simulink model "METI_Thermal_ver01_Jmaab_2018b_Intg_Mref"  (R2018b)
settings: Solver=ode8  StartTime=0  StopTime=end_time  FixedStep=sampling_time  RelTol=1e-3
PreLoadFcn:
  | %init_setting;
values from neighbouring files (symbols this model uses):
  degC2K = 273.15    [METI_TRAMI_Thermal_ver01_Jmaab_PreLoad.m]    (also in init_setting_METI.m)
  K2degC = -273.15    [METI_TRAMI_Thermal_ver01_Jmaab_PreLoad.m]    (also in init_setting_METI.m)
  sampling_time = 0.0025    [METI_TRAMI_Thermal_ver01_Jmaab_PreLoad.m]
undefined symbols (not defined in the file or in its folder): ACC_D_Gain, ACC_I_Gain, ACC_P_Gain, ALT_CNT_ALT_OFF_RPM_HYS_rpm, ALT_CNT_ALT_ON_RPM_HYS_rpm, ALT_CNT_Alter_V_BASE_V, ALT_CNT_Alter_V_Kaisei_V, ALT_CNT_flag_disable_kaisei, ALT_CNT_V_Battely_Kudo_V, ALT_PNT_ALT_GDCurrent_A, ALT_PNT_ALT_GDVolt_V, ALT_PNT_Alter_limit_Current_V_table, ALT_PNT_Alter_limit_Current_V_table_x_rpm, ALT_PNT_Alter_trq_Nm_map, ALT_PNT_Alter_trq_Nm_map_x_rpm, ALT_PNT_Alter_trq_Nm_map_y_Current_A, ALT_PNT_Alter_trq_Nm_map_z_Volt_tgt_V, ALT_PNT_eta_pulley_alt, ALT_PNT_Gain_Alt_v_del, ALT_PNT_ratio_pulley_alt, ALT_PNT_Tau_Alternator_V_tgt_s, ALT_PNT_trq_alter_output_LL_Nm, BK_PNT_Pow_UL, BK_PNT_Tau_brake, Brk_LL, Brk_PGain, Brk_UL, BT_PNT_Lo_Capa_lo_batt_F, BT_PNT_Lo_ocv_SOC_lo_batt_OCV_V_table, BT_PNT_Lo_ocv_SOC_lo_batt_OCV_V_table_x_SOC, BT_PNT_Lo_R_lo_batt_ohm, BT_PNT_Lo_SOC_MAX_lo_batt, BT_PNT_Lo_SOC_MIN_lo_batt, BT_PNT_Lo_SOC_START_lo_batt, BT_PNT_Lo_V_start_ocv, DF_PNT_DF_gear, DF_PNT_Outtemp_degC, Driver_Brake_Const1, Driver_Brake_Const3, Driver_Brake_Switch_Const2, Driver_Brk_sh, drivmode_ACC, drivmode_CONST, drivmode_GensokuKaisei, drivmode_GensokuRikko, drivmode_STOP, EL_PNT_R_bodyelec_lo_ohm, ENG_CNT_acc_idlestop, ENG_CNT_Accel_LL, ENG_CNT_Accel_UL, ENG_CNT_brak_idlestop, ENG_CNT_flag_idle_stop_exe, ENG_CNT_gain_p_per_isc, ENG_CNT_IdleSpeed, ENG_CNT_IdleSpeed_Const, ENG_CNT_IdleStop_flag_const, ENG_CNT_omg_eng_fuelcut_rpm, ENG_CNT_per_isc_max, ENG_CNT_per_isc_min, ENG_CNT_per_throttle_fuelcut ... (+82)
libraries: METI_Lib_vehicle_model x18, simulink x3, AZAPA_Lib_vehicle_model x1
(part 3 of 3)

== system METI_Thermal_ver01_Jmaab_2018b_Intg_Mref/Vehicle/CNT/ENG_CNT/ENG_Cntrl/Starter ==
  note: サンプリング時間
  note: 時間リセット
  note: アイドリングフラグがON→OFFに
      | 切り替わり時スターターON開始
  note: スタータ開始時間
  note: スタータ開始時間から
      | ある時間超えたらOFF
  note: アイドリングフラグがON→OFFに切り替わり時スターターON開始.ある時間を超えたらOFF
  flag_idlestop : Inport
  n_eng_rpm : Inport  Port=2
  Constant2 : Constant  Value=ENG_CNT_Starter_timer_Const_s
  Constant4 : Constant  Value=sampling_time
  Constant5 : Constant  Value=0
  Constant6 : Constant  Value=OFF
  Constant7 : Constant  Value=ON
  IdleSpeed : Constant  Value=ENG_CNT_IdleSpeed_Const/2
  Logical Operator : Logic  Inputs=3  AllPortsSameDT=off  OutDataTypeStr=boolean
  Logical Operator1 : Logic  Operator=NOT  AllPortsSameDT=off  OutDataTypeStr=boolean
  Memory : Memory  InitialCondition=1000
  Memory1 : Memory  InheritSampleTime=on
  Relational Operator1 : RelationalOperator  Operator=<=  OutDataTypeStr=boolean  RndMeth=Nearest
  Relational Operator2 : RelationalOperator  Operator=<  OutDataTypeStr=boolean  RndMeth=Nearest
  Sum5 : Sum  Inputs=|++
  Switch3 : Switch  Criteria=u2 > Threshold  Threshold=0.5
  Switch4 : Switch  Criteria=u2 > Threshold  Threshold=0.5
  flag_ON_Starter : Outport
  wires:
  Switch4/1 -> flag_ON_Starter/1
  Memory/1 -> Sum5/2
  Constant4/1 -> Sum5/1
  Constant5/1 -> Switch3/1
  Sum5/1 -> Switch3/3
  Switch3/1 -> Relational Operator1/1, Memory/1
  Memory1/1 -> Logical Operator/2
  Logical Operator1/1 -> Logical Operator/1
  flag_idlestop/1 -> Memory1/1, Logical Operator1/1
  Logical Operator/1 -> Switch3/2
  Constant2/1 -> Relational Operator1/2
  Relational Operator1/1 -> Switch4/2
  Constant7/1 -> Switch4/1
  Constant6/1 -> Switch4/3
  n_eng_rpm/1 -> Relational Operator2/1
  IdleSpeed/1 -> Relational Operator2/2
  Relational Operator2/1 -> Logical Operator/3

== system METI_Thermal_ver01_Jmaab_2018b_Intg_Mref/Vehicle/CNT/ENG_CNT/ENG_Cntrl/Water_Pump_Control ==
  T_ENGTH_PNT_Coolant_dC : Inport
  1-D Lookup Table1 : Lookup_n-D  NumberOfTableDimensions=1  BreakpointsForDimension1=ENG_CNT_V_Water_Pump_x_T_Coolant  BeginIndexSearchUsingPreviousIndexResult=on  Table=ENG_CNT_V_Water_Pump_V  InternalRulePriority=Speed  RndMeth=Simplest  InputSameDT=on
  V_ENG_PNT_WP_V : Outport
  wires:
  T_ENGTH_PNT_Coolant_dC/1 -> 1-D Lookup Table1/1
  1-D Lookup Table1/1 -> V_ENG_PNT_WP_V/1

== system METI_Thermal_ver01_Jmaab_2018b_Intg_Mref/Vehicle/ENG_PNT/ENG_Plant/Cal_FuelComsunption/Not_cal1 ==
  In1 : Inport
  Constant : Constant  Value=0
  Constant1 : Constant
  Switch : Switch  Criteria=u2 > Threshold  Threshold=0.5
  Out1 : Outport
  wires:
  Constant1/1 -> Switch/3
  Constant/1 -> Switch/1
  Switch/1 -> Out1/1
  In1/1 -> Switch/2

== system METI_Thermal_ver01_Jmaab_2018b_Intg_Mref/Vehicle/ENG_PNT/ENG_Plant/Cal_FuelComsunption/Not_cal2 ==
  In1 : Inport
  Constant : Constant  Value=0
  Constant1 : Constant
  Switch : Switch  Criteria=u2 > Threshold  Threshold=0.5
  Out1 : Outport
  wires:
  In1/1 -> Switch/2
  Switch/1 -> Out1/1
  Constant/1 -> Switch/1
  Constant1/1 -> Switch/3

== system METI_Thermal_ver01_Jmaab_2018b_Intg_Mref/Vehicle/ENG_PNT/ENG_Plant/Cal_trq_ENG_jiku/Not_cal ==
  In1 : Inport
  Constant : Constant  Value=0
  Constant1 : Constant
  Switch : Switch  Criteria=u2 > Threshold  Threshold=0.5
  Out1 : Outport
  wires:
  In1/1 -> Switch/2
  Switch/1 -> Out1/1
  Constant/1 -> Switch/1
  Constant1/1 -> Switch/3

== system METI_Thermal_ver01_Jmaab_2018b_Intg_Mref/Vehicle/ENG_PNT/ENG_Plant/Cal_trq_ENG_jiku/Not_cal1 ==
  In1 : Inport
  Constant : Constant  Value=0
  Constant1 : Constant
  Switch : Switch  Criteria=u2 > Threshold  Threshold=0.5
  Out1 : Outport
  wires:
  Constant1/1 -> Switch/3
  Constant/1 -> Switch/1
  Switch/1 -> Out1/1
  In1/1 -> Switch/2

== system METI_Thermal_ver01_Jmaab_2018b_Intg_Mref/Vehicle/PTTH/ENGTH_PNT/ENGTH/Coolant_Heat_Capacity ==
  PHI_Coolant4_W : Inport
  PHI_Coolant1_W : Inport  Port=2
  PHI_Coolant3_W : Inport  Port=3
  PHI_Coolant2_W : Inport  Port=4
  Add : Sum  Inputs=++++
  Add1 : Sum
  Constant : Constant  Value=ENG_PNT_Coolant_Heat_Capa_JpK
  Constant1 : Constant  Value=ENG_PNT_Coolant_Temp_ini_degC
  Divide : Product  Inputs=/*
  Integrator : Integrator
  degC->K : Subsystem
  T_Coolant1_K : Outport
  T_Coolant4_K : Outport  Port=2
  T_Coolant2_K : Outport  Port=3
  T_Coolant3_K : Outport  Port=4
  wires:
  PHI_Coolant2_W/1 -> Add/4
  PHI_Coolant1_W/1 -> Add/1
  Constant/1 -> Divide/1
  Add/1 -> Divide/2
  Divide/1 -> Integrator/1
  Integrator/1 -> Add1/2
  Add1/1 -> T_Coolant3_K/1, T_Coolant2_K/1, T_Coolant4_K/1, T_Coolant1_K/1
  PHI_Coolant3_W/1 -> Add/2
  PHI_Coolant4_W/1 -> Add/3
  degC->K/1(K) -> Add1/1
  Constant1/1 -> degC->K/1(degC)

== system METI_Thermal_ver01_Jmaab_2018b_Intg_Mref/Vehicle/PTTH/ENGTH_PNT/ENGTH/Cylinder_Head2Coolant_Heat_Resistance ==
  T_Coolant_Resi1_K : Inport
  Qv_Coolant_m3ps : Inport  Port=2
  T_Cylinder_Head_Resi2_K : Inport  Port=3
  1-D Lookup Table : Lookup_n-D  NumberOfTableDimensions=1  BreakpointsForDimension1=ENG_PNT_Cylinder_Head2Coolant_Heat_Resi_x_qv_Coolant  Table=ENG_PNT_Cylinder_Head2Coolant_Heat_Resi_KpW  InternalRulePriority=Speed  RndMeth=Simplest  InputSameDT=on
  Add : Sum  Inputs=+-
  Divide : Product  Inputs=*/
  Gain : Gain  Gain=-1
  Gain1 : Gain
  PHI_Coolant_Resi1_W : Outport
  PHI_Cylinder_Head_Resi2_W : Outport  Port=2
  wires:
  T_Cylinder_Head_Resi2_K/1 -> Add/1
  T_Coolant_Resi1_K/1 -> Add/2
  1-D Lookup Table/1 -> Divide/2
  Add/1 -> Divide/1
  Divide/1 -> Gain/1, Gain1/1
  Gain/1 -> PHI_Cylinder_Head_Resi2_W/1
  Gain1/1 -> PHI_Coolant_Resi1_W/1
  Qv_Coolant_m3ps/1 -> 1-D Lookup Table/1

== system METI_Thermal_ver01_Jmaab_2018b_Intg_Mref/Vehicle/PTTH/ENGTH_PNT/ENGTH/ENGBlock2Air_Heat_Resistance ==
  T_ENGBlock_Resi3_K : Inport
  T_ENG_Air_Resi1_K : Inport  Port=2
  Add : Sum  Inputs=+-
  Constant : Constant  Value=ENG_PNT_ENGBlock2ENGAir_Heat_Resi_KpW
  Divide : Product  Inputs=*/
  Gain : Gain  Gain=-1
  Gain1 : Gain
  PHI_ENGBlock_Resi3_W : Outport
  PHI_ENG_Air_Resi1_W : Outport  Port=2
  wires:
  Constant/1 -> Divide/2
  Add/1 -> Divide/1
  Divide/1 -> Gain1/1, Gain/1
  Gain/1 -> PHI_ENGBlock_Resi3_W/1
  T_ENGBlock_Resi3_K/1 -> Add/1
  T_ENG_Air_Resi1_K/1 -> Add/2
  Gain1/1 -> PHI_ENG_Air_Resi1_W/1

== system METI_Thermal_ver01_Jmaab_2018b_Intg_Mref/Vehicle/PTTH/ENGTH_PNT/ENGTH/ENGBlock2Coolant_Heat_Resistance ==
  T_Coolant_Resi4_K : Inport
  T_ENGBlock_Resi1_K : Inport  Port=2
  Add : Sum  Inputs=+-
  Constant : Constant  Value=ENG_PNT_Coolant2ENGBlock_Heat_Resi_KpW
  Divide : Product  Inputs=*/
  Gain : Gain  Gain=-1
  Gain1 : Gain
  PHI_Coolant_Resi4_W : Outport
  PHI_ENGBlock_Resi1_W : Outport  Port=2
  wires:
  Constant/1 -> Divide/2
  Add/1 -> Divide/1
  Divide/1 -> Gain1/1, Gain/1
  Gain/1 -> PHI_Coolant_Resi4_W/1
  T_Coolant_Resi4_K/1 -> Add/1
  T_ENGBlock_Resi1_K/1 -> Add/2
  Gain1/1 -> PHI_ENGBlock_Resi1_W/1

== system METI_Thermal_ver01_Jmaab_2018b_Intg_Mref/Vehicle/PTTH/ENGTH_PNT/ENGTH/ENGBlock_Heat_Capacity ==
  PHI_ENGBlock3_W : Inport
  PHI_ENGBlock1_W : Inport  Port=2
  PHI_ENGBlock2_W : Inport  Port=3
  Add : Sum  Inputs=+++
  Add1 : Sum
  Constant : Constant  Value=ENG_PNT_ENGBlock_Heat_Capa_JpK
  Constant1 : Constant  Value=ENG_PNT_ENGBlock_Temp_ini_degC
  Divide : Product  Inputs=/*
  Integrator : Integrator
  degC->K : Subsystem
  T_ENGBlock3_K : Outport
  T_ENGBlock2_K : Outport  Port=2
  T_ENGBlock1_K : Outport  Port=3
  wires:
  PHI_ENGBlock2_W/1 -> Add/3
  PHI_ENGBlock1_W/1 -> Add/1
  Constant/1 -> Divide/1
  Add/1 -> Divide/2
  Divide/1 -> Integrator/1
  Integrator/1 -> Add1/2
  Add1/1 -> T_ENGBlock2_K/1, T_ENGBlock1_K/1, T_ENGBlock3_K/1
  PHI_ENGBlock3_W/1 -> Add/2
  Constant1/1 -> degC->K/1(degC)
  degC->K/1(K) -> Add1/1

== system METI_Thermal_ver01_Jmaab_2018b_Intg_Mref/Vehicle/PTTH/ENGTH_PNT/ENGTH/ENGOil2Coolant_Heat_Resistance ==
  T_ENGOil_Resi2_K : Inport
  T_Coolant_Resi3_K : Inport  Port=2
  Add : Sum  Inputs=+-
  Constant : Constant  Value=ENG_PNT_ENGOil2Coolant_Heat_Resi_KpW
  Divide : Product  Inputs=*/
  Gain : Gain  Gain=-1
  Gain1 : Gain
  PHI_ENGOil_Resi2_W : Outport
  PHI_Coolant_Resi3_W : Outport  Port=2
  wires:
  T_ENGOil_Resi2_K/1 -> Add/1
  T_Coolant_Resi3_K/1 -> Add/2
  Constant/1 -> Divide/2
  Add/1 -> Divide/1
  Divide/1 -> Gain/1, Gain1/1
  Gain/1 -> PHI_ENGOil_Resi2_W/1
  Gain1/1 -> PHI_Coolant_Resi3_W/1

== system METI_Thermal_ver01_Jmaab_2018b_Intg_Mref/Vehicle/PTTH/ENGTH_PNT/ENGTH/ENGOil_Heat_Capacity ==
  PHI_ENGOil2_W : Inport
  PHI_ENGOil1_W : Inport  Port=2
  Add : Sum
  Add1 : Sum
  Constant : Constant  Value=ENG_PNT_ENGOil_Heat_Capa_JpK
  Constant1 : Constant  Value=ENG_PNT_ENGOil_Temp_ini_degC
  Divide : Product  Inputs=/*
  Integrator : Integrator
  degC->K : Subsystem
  T_ENGOil2_K : Outport
  T_ENGOil1_K : Outport  Port=2
  wires:
  PHI_ENGOil2_W/1 -> Add/2
  PHI_ENGOil1_W/1 -> Add/1
  Constant/1 -> Divide/1
  Add/1 -> Divide/2
  Divide/1 -> Integrator/1
  Integrator/1 -> Add1/2
  Add1/1 -> T_ENGOil2_K/1, T_ENGOil1_K/1
  Constant1/1 -> degC->K/1(degC)
  degC->K/1(K) -> Add1/1

== system METI_Thermal_ver01_Jmaab_2018b_Intg_Mref/Vehicle/PTTH/ENGTH_PNT/ENGTH/ENGOil_Heat_Capacity1 ==
  PHI_Cylinder_Head1_W : Inport
  PHI_Cylinder_Head2_W : Inport  Port=2
  Add : Sum
  Add1 : Sum
  Constant : Constant  Value=ENG_PNT_Cylinder_Head_Heat_Capa_JpK
  Constant1 : Constant  Value=ENG_PNT_Cylinder_Head_Temp_ini_degC
  Divide : Product  Inputs=/*
  Integrator : Integrator
  degC->K : Subsystem
  T_Cylinder_Head1_K : Outport
  T_Cylinder_Head2_K : Outport  Port=2
  wires:
  PHI_Cylinder_Head2_W/1 -> Add/2
  PHI_Cylinder_Head1_W/1 -> Add/1
  Constant/1 -> Divide/1
  Add/1 -> Divide/2
  Divide/1 -> Integrator/1
  Integrator/1 -> Add1/2
  Add1/1 -> T_Cylinder_Head2_K/1, T_Cylinder_Head1_K/1
  Constant1/1 -> degC->K/1(degC)
  degC->K/1(K) -> Add1/1

== system METI_Thermal_ver01_Jmaab_2018b_Intg_Mref/Vehicle/PTTH/ENGTH_PNT/ENGTH/Water_Pump ==
  ENG_PNT_Voltage_WP_V : Inport
  1-D Lookup Table : Lookup_n-D  NumberOfTableDimensions=1  BreakpointsForDimension1=ENG_PNT_Qv_Water_Pump_x_V_WP  Table=ENG_PNT_Qv_Water_Pump_m3ps  InternalRulePriority=Speed  RndMeth=Simplest  InputSameDT=on
  Qv_Coolant_m3ps : Outport
  wires:
  ENG_PNT_Voltage_WP_V/1 -> 1-D Lookup Table/1
  1-D Lookup Table/1 -> Qv_Coolant_m3ps/1

== system METI_Thermal_ver01_Jmaab_2018b_Intg_Mref/Vehicle/PTTH/RDTH_PNT/RDTH/ENGBlock2Coolant_Heat_Resistance ==
  T_RDCoolant_Resi1_K : Inport
  T_Thermostat_Resi1_K : Inport  Port=2
  1-D Lookup Table : Lookup_n-D  NumberOfTableDimensions=1  BreakpointsForDimension1=RD_PNT_Thermostat_Heat_Resi_KpW_T_Coolant  Table=RD_PNT_Thermostat_Heat_Resi_KpW  InternalRulePriority=Speed  RndMeth=Simplest  InputSameDT=on
  Add : Sum  Inputs=+-
  Divide : Product  Inputs=*/
  Gain : Gain  Gain=-1
  Gain1 : Gain
  K->degC : Subsystem
  PHI_RDCoolant_Resi1_W : Outport
  PHI_Thermostat_Resi1_W : Outport  Port=2
  tag scope: RD_PNT_Thermostat_Heat_Resi_KpW=global
  wires:
  Add/1 -> Divide/1
  Divide/1 -> Gain/1, Gain1/1
  Gain/1 -> PHI_Thermostat_Resi1_W/1
  T_Thermostat_Resi1_K/1 -> Add/1, K->degC/1(K)
  T_RDCoolant_Resi1_K/1 -> Add/2
  Gain1/1 -> PHI_RDCoolant_Resi1_W/1
  K->degC/1(degC) -> 1-D Lookup Table/1
  1-D Lookup Table/1 -> [RD_PNT_Thermostat_Heat_Resi_KpW], Divide/2

== system METI_Thermal_ver01_Jmaab_2018b_Intg_Mref/Vehicle/PTTH/RDTH_PNT/RDTH/RDCoolant2Air_Heat_Resistance ==
  T_RD_Air_Resi_K : Inport
  "RD_PNT_RDCore_Heat_Resi_KpW " : Inport  Port=2
  T_RDCoolant_Resi2_K : Inport  Port=3
  Add : Sum  Inputs=+-
  Divide : Product  Inputs=*/
  Gain : Gain  Gain=-1
  Gain1 : Gain
  PHI_RD_Air_Resi1_W : Outport
  PHI_RDCoolant_Resi2_W : Outport  Port=2
  wires:
  "RD_PNT_RDCore_Heat_Resi_KpW "/1 -> Divide/2
  Add/1 -> Divide/1
  Divide/1 -> Gain/1, Gain1/1
  Gain/1 -> PHI_RDCoolant_Resi2_W/1
  T_RDCoolant_Resi2_K/1 -> Add/1
  T_RD_Air_Resi_K/1 -> Add/2
  Gain1/1 -> PHI_RD_Air_Resi1_W/1

== system METI_Thermal_ver01_Jmaab_2018b_Intg_Mref/Vehicle/PTTH/RDTH_PNT/RDTH/RDCoolant_Heat_Capacity ==
  PHI_RDCoolant1_W : Inport
  PHI_RDCoolant2_W : Inport  Port=2
  Add : Sum
  Add1 : Sum
  Constant : Constant  Value=RD_PNT_RDCoolant_Heat_Capa_JpK
  Constant1 : Constant  Value=RD_PNT_RDCoolant_Temp_ini_degC
  Divide : Product  Inputs=/*
  Integrator : Integrator
  degC->K : Subsystem
  T_RDCoolant1_K : Outport
  T_RDCoolant2_K : Outport  Port=2
  wires:
  PHI_RDCoolant2_W/1 -> Add/2
  PHI_RDCoolant1_W/1 -> Add/1
  Constant/1 -> Divide/1
  Add/1 -> Divide/2
  Divide/1 -> Integrator/1
  Integrator/1 -> Add1/2
  Add1/1 -> T_RDCoolant2_K/1, T_RDCoolant1_K/1
  Constant1/1 -> degC->K/1(degC)
  degC->K/1(K) -> Add1/1

== system METI_Thermal_ver01_Jmaab_2018b_Intg_Mref/Vehicle/PTTH/RDTH_PNT/RDTH/RD_Core_Heat_Resi_Calc ==
  note: ラジエターファンの動作で
      | 発生する風速
  note: 車両の走行によって
      | ラジエターグリルに発生する風速
  note: ラジエターファンの動作で
      | ラジエターコアに当たる風量
  note: 車両の走行によって
      | ラジエターコアに当たる風量
  RD_PNT_Voltage_RDFan_V : Inport
  v_VL_PNT_kmph : Inport  Port=2
  1-D Lookup Table : Lookup_n-D  NumberOfTableDimensions=1  BreakpointsForDimension1=RD_PNT_RDCore_Heat_Resi_KpW_x_Wind_m3ps  Table=RD_PNT_RDCore_Heat_Resi_KpW  InternalRulePriority=Speed  RndMeth=Simplest  InputSameDT=on
  1-D Lookup Table1 : Lookup_n-D  NumberOfTableDimensions=1  BreakpointsForDimension1=RD_PNT_v_RDFan_Wind_vel_mps_x_V_RDFan  Table=RD_PNT_v_RDFan_Wind_vel_mps  InternalRulePriority=Speed  RndMeth=Simplest  InputSameDT=on
  Abs : Abs
  Add : Sum
  Constant : Constant  Value=RD_PNT_RDFan_area_m2
  Constant1 : Constant  Value=RD_PNT_RDGrill_area_m2
  Product : Product
  Product1 : Product
  gain1 : Gain  Gain=kmph2mps
  "RD_PNT_RDCore_Heat_Resi_KpW " : Outport
  wires:
  RD_PNT_Voltage_RDFan_V/1 -> 1-D Lookup Table1/1
  Constant/1 -> Product/2
  v_VL_PNT_kmph/1 -> gain1/1
  Constant1/1 -> Product1/2
  Product/1 -> Add/1
  Product1/1 -> Add/2
  Add/1 -> Abs/1
  1-D Lookup Table/1 -> "RD_PNT_RDCore_Heat_Resi_KpW "/1
  Abs/1 -> 1-D Lookup Table/1
  1-D Lookup Table1/1 -> Product/1
  gain1/1 -> Product1/1

== system METI_Thermal_ver01_Jmaab_2018b_Intg_Mref/Vehicle/CNT/ENG_CNT/ENG_Cntrl/Caliculate_Idle_Speed/Subsystem ==
  del_omg_engine : Inport
  flag_idle_fb : Inport  Port=2
  Gain : Gain  Gain=ENG_CNT_gain_p_per_isc
  Logical Operator1 : Logic  Operator=NOT  AllPortsSameDT=off  OutDataTypeStr=boolean
  Memory : Memory  InitialCondition=4
  Saturation : Saturate  UpperLimit=ENG_CNT_per_isc_max  LowerLimit=ENG_CNT_per_isc_min
  Switch : Switch  Criteria=u2 > Threshold  Threshold=0.5
  per_isc_[%] : Outport
  wires:
  Switch/1 -> Saturation/1
  flag_idle_fb/1 -> Logical Operator1/1
  Gain/1 -> Switch/3
  Memory/1 -> Switch/1
  Saturation/1 -> per_isc_[%]/1, Memory/1
  del_omg_engine/1 -> Gain/1
  Logical Operator1/1 -> Switch/2

== system METI_Thermal_ver01_Jmaab_2018b_Intg_Mref/Vehicle/CNT/ENG_CNT/ENG_Cntrl/Caliculate_Idle_Speed/Subsystem1 ==
  note: アイドル回転数時のFB
  omg_tgt_idle : Inport
  n_eng_rpm : Inport  Port=2
  per_throttle_base : Inport  Port=3
  flag_Lockup : Inport  Port=4
  flag_IdleStop : Inport  Port=5
  Logical Operator : Logic  Operator=OR  AllPortsSameDT=off  OutDataTypeStr=boolean
  Logical Operator1 : Logic  Operator=NOT  AllPortsSameDT=off  OutDataTypeStr=boolean
  Logical Operator2 : Logic  Inputs=3  AllPortsSameDT=off  OutDataTypeStr=boolean
  Logical Operator3 : Logic  Operator=NOT  AllPortsSameDT=off  OutDataTypeStr=boolean
  Logical Operator4 : Logic  Operator=NOT  AllPortsSameDT=off  OutDataTypeStr=boolean
  Logical Operator5 : Logic  AllPortsSameDT=off  OutDataTypeStr=boolean
  Relational Operator : RelationalOperator  Operator=<  OutDataTypeStr=boolean  RndMeth=Nearest
  Relational Operator2 : RelationalOperator  Operator=>  OutDataTypeStr=boolean  RndMeth=Nearest
  per_throttle_isc_fb : Constant  Value=ENG_CNT_per_throttle_isc_fb
  flag_idle_fb : Outport
  wires:
  per_throttle_base/1 -> Relational Operator/1
  per_throttle_isc_fb/1 -> Relational Operator/2
  Relational Operator2/1 -> Logical Operator2/1
  Relational Operator/1 -> Logical Operator1/1, Logical Operator5/1
  Logical Operator1/1 -> Logical Operator2/2
  Logical Operator5/1 -> Logical Operator/2
  flag_Lockup/1 -> Logical Operator3/1
  Logical Operator3/1 -> Logical Operator2/3
  Logical Operator2/1 -> Logical Operator/1
  omg_tgt_idle/1 -> Relational Operator2/1
  n_eng_rpm/1 -> Relational Operator2/2
  flag_IdleStop/1 -> Logical Operator4/1
  Logical Operator4/1 -> Logical Operator5/2
  Logical Operator/1 -> flag_idle_fb/1

== system METI_Thermal_ver01_Jmaab_2018b_Intg_Mref/Vehicle/PTTH/ENGTH_PNT/ENGTH/Coolant_Heat_Capacity/degC->K ==
  degC : Inport
  Constant2 : Constant  Value=degC2K
  Sum : Sum  Inputs=++|
  K : Outport
  wires:
  degC/1 -> Sum/2
  Constant2/1 -> Sum/1
  Sum/1 -> K/1

== system METI_Thermal_ver01_Jmaab_2018b_Intg_Mref/Vehicle/PTTH/ENGTH_PNT/ENGTH/ENGBlock_Heat_Capacity/degC->K ==
  degC : Inport
  Constant2 : Constant  Value=degC2K
  Sum : Sum  Inputs=++|
  K : Outport
  wires:
  degC/1 -> Sum/2
  Constant2/1 -> Sum/1
  Sum/1 -> K/1

== system METI_Thermal_ver01_Jmaab_2018b_Intg_Mref/Vehicle/PTTH/ENGTH_PNT/ENGTH/ENGOil_Heat_Capacity/degC->K ==
  degC : Inport
  Constant2 : Constant  Value=degC2K
  Sum : Sum  Inputs=++|
  K : Outport
  wires:
  degC/1 -> Sum/2
  Constant2/1 -> Sum/1
  Sum/1 -> K/1

== system METI_Thermal_ver01_Jmaab_2018b_Intg_Mref/Vehicle/PTTH/ENGTH_PNT/ENGTH/ENGOil_Heat_Capacity1/degC->K ==
  degC : Inport
  Constant2 : Constant  Value=degC2K
  Sum : Sum  Inputs=++|
  K : Outport
  wires:
  degC/1 -> Sum/2
  Constant2/1 -> Sum/1
  Sum/1 -> K/1

== system METI_Thermal_ver01_Jmaab_2018b_Intg_Mref/Vehicle/PTTH/RDTH_PNT/RDTH/ENGBlock2Coolant_Heat_Resistance/K->degC ==
  K : Inport
  Constant2 : Constant  Value=K2degC
  Sum : Sum  Inputs=++|
  degC : Outport
  wires:
  K/1 -> Sum/2
  Constant2/1 -> Sum/1
  Sum/1 -> degC/1

== system METI_Thermal_ver01_Jmaab_2018b_Intg_Mref/Vehicle/PTTH/RDTH_PNT/RDTH/RDCoolant_Heat_Capacity/degC->K ==
  degC : Inport
  Constant2 : Constant  Value=degC2K
  Sum : Sum  Inputs=++|
  K : Outport
  wires:
  degC/1 -> Sum/2
  Constant2/1 -> Sum/1
  Sum/1 -> K/1
